simulink subsystem "thermal_subsystem_controller"  (R2023a)
settings: Solver=VariableStepAuto  StartTime=0.0  StopTime=10.0  RelTol=1e-3
undefined symbols (not defined in the file or in its folder): b_auxTCP_ACT, b_TCP_ACT, b_TCV_ACT, struct_auxTCP_ACT, struct_TCP_ACT, struct_TCV_ACT, struct_ThermalAct
libraries: simulink x4, eeGeneralControl x4, slpidlib x2
settings Model: Creator=daniel.harlander  LastModifiedBy=adrian.taveras
settings OptimizationCC: ReuseModelBlockBuffer=off

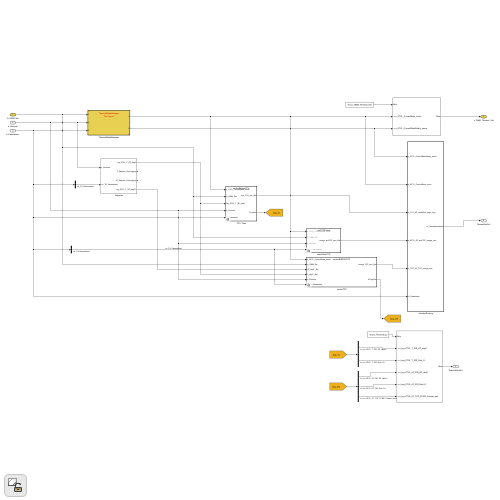
[thumbnail: Simulink's stored preview of the top-level diagram]
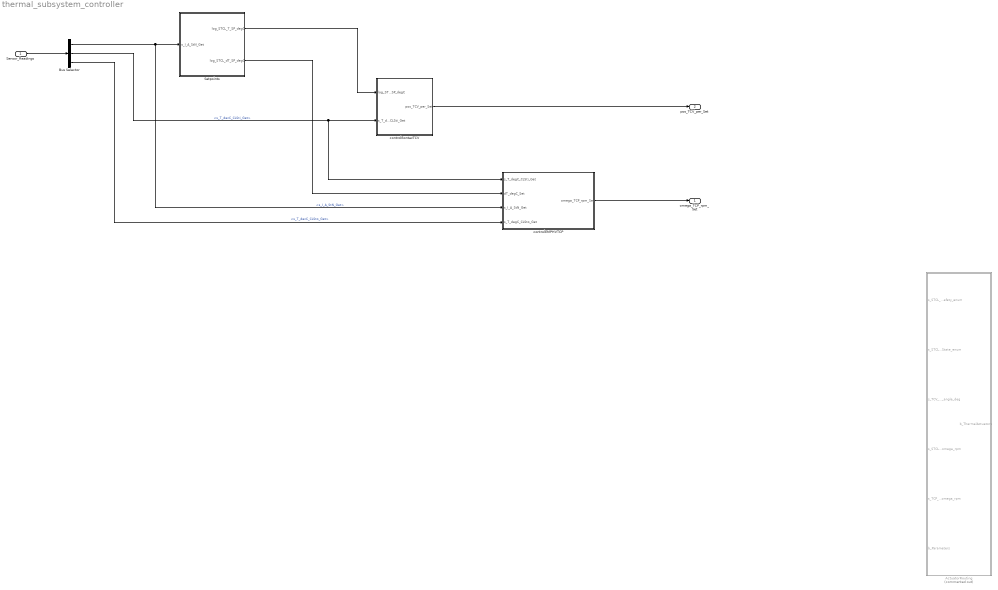
== system thermal_subsystem_controller ==
  Sensor_Readings : Inport
  ActuatorRouting : Subsystem  Commented=on  TreatAsAtomicUnit=on
      settings: RTWFcnNameOpts=Use subsystem name  RTWFileNameOpts=Use subsystem name
  Bus Selector : BusSelector  OutputSignals=s_I_A_StN_Get,s_T_decC_CLSti_Get,s_T_decC_CLSto_Get
  Setpoints : Subsystem
  controlBontazTCV : Subsystem  TreatAsAtomicUnit=on  VariantControl=variantConfig.TCV == VARIANT_TCV.BontazCAN
      settings: RTWFcnNameOpts=Use subsystem name  RTWFileNameOpts=Use subsystem name
  controlEMPHVTCP : Subsystem  TreatAsAtomicUnit=on  VariantControl=variantConfig.TCP == VARIANT_TCP.HVPump
  omega_TCP_rpm_Set : Outport
  pos_TCV_per_Set : Outport  Port=2
  wires:
  Setpoints/1(log_STCL_T_SP_degC) -> controlBontazTCV/1(log_STCL_T_SP_degC)
  Setpoints/2(log_STCL_dT_SP_degC) -> controlEMPHVTCP/2(dT_degC_Set)
  controlEMPHVTCP/1(omega_TCP_rpm_Set) -> omega_TCP_rpm_Set/1
  Sensor_Readings/1 -> Bus Selector/1
  Bus Selector/1 -> Setpoints/1(s_I_A_StN_Get), controlEMPHVTCP/3(s_I_A_StN_Get)  "<s_I_A_StN_Get>"
  Bus Selector/2 -> controlBontazTCV/2(s_T_decC_CLSti_Get), controlEMPHVTCP/1(s_T_degC_CLSti_Get)  "<s_T_decC_CLSti_Get>"
  Bus Selector/3 -> controlEMPHVTCP/4(s_T_degC_CLSto_Get)  "<s_T_decC_CLSto_Get>"
  controlBontazTCV/1(pos_TCV_per_Set) -> pos_TCV_per_Set/1

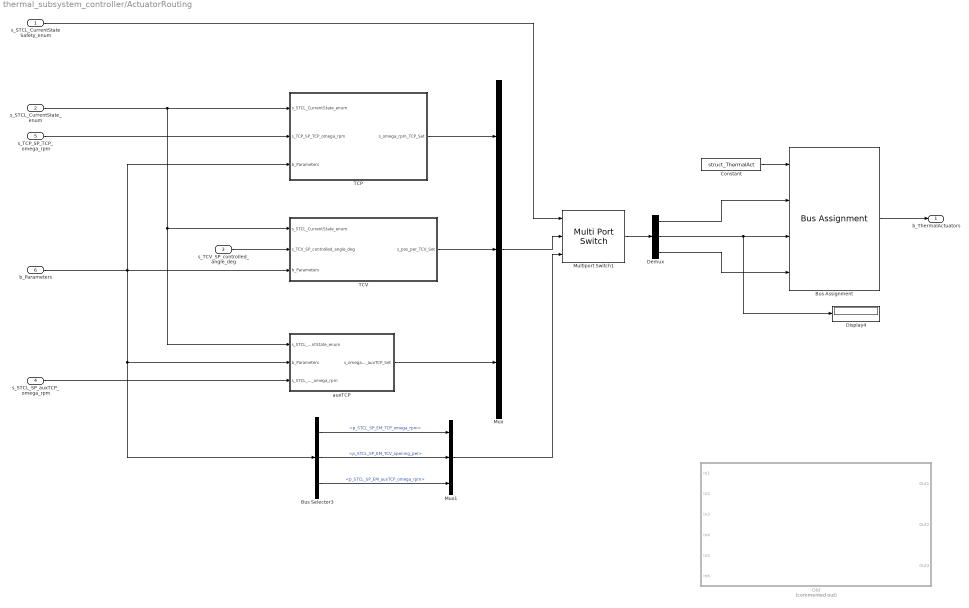
== system thermal_subsystem_controller/ActuatorRouting ==
  s_STCL_CurrentStateSafety_enum : Inport
  s_STCL_CurrentState_enum : Inport  Port=2
  s_TCV_SP_controlled_angle_deg : Inport  Port=3
  s_STCL_SP_auxTCP_omega_rpm : Inport  Port=4
  s_TCP_SP_TCP_omega_rpm : Inport  Port=5
  "b_Parameters  " : Inport  Port=6  OutDataTypeStr=Bus: Parameters
  Bus Assignment : BusAssignment  AssignedSignals=b_TCP_ACT.s_omega_rpm_TCP_Set,b_TCV_ACT.s_pos_per_TCV_Set,b_auxTCP_ACT.s_omega_rpm_auxTCP_Set
  Bus Selector3 : BusSelector  OutputSignals=b_TH_Parameters.b_STCL_Parameters.p_STCL_SP_EM_TCP_omega_rpm,b_TH_Parameters.b_STCL_Parameters.p_STCL_SP_EM_TCV_opening_per,b_TH_Parameters.b_STCL_Parameters.p_STCL_SP_EM_auxTCP_omega_rpm
  Constant : Constant  Value=struct_ThermalAct  OutDataTypeStr=Bus: ThermalAct
  Demux : Demux  Outputs=3
  Display4 : Display
  Multiport Switch1 : MultiPortSwitch  DataPortOrder=Specify indices  DataPortIndices={STCL_STATE_SAFETY.Safe, STCL_STATE_SAFETY.ESD_Off}  SaturateOnIntegerOverflow=off  InputSameDT=off
  Mux : Mux  Inputs=3
  Mux1 : Mux  Inputs=3
  Old : Subsystem  Commented=on
  TCP : Subsystem
  TCV : Subsystem
  auxTCP : Subsystem
  b_ThermalActuators : Outport
  wires:
  TCP/1(s_omega_rpm_TCP_Set) -> Mux/1
  s_TCP_SP_TCP_omega_rpm/1 -> TCP/2(s_TCP_SP_TCP_omega_rpm)
  TCV/1(s_pos_per_TCV_Set) -> Mux/2
  s_TCV_SP_controlled_angle_deg/1 -> TCV/2(s_TCV_SP_controlled_angle_deg)
  auxTCP/1(s_omega_rpm_auxTCP_Set) -> Mux/3
  s_STCL_SP_auxTCP_omega_rpm/1 -> auxTCP/3(s_STCL_SP_auxTCP_omega_rpm)
  Demux/3 -> Bus Assignment/4
  Demux/1 -> Bus Assignment/2
  Demux/2 -> Bus Assignment/3, Display4/1
  s_STCL_CurrentStateSafety_enum/1 -> Multiport Switch1/1
  Constant/1 -> Bus Assignment/1
  Bus Assignment/1 -> b_ThermalActuators/1
  s_STCL_CurrentState_enum/1 -> TCP/1(s_STCL_CurrentState_enum), TCV/1(s_STCL_CurrentState_enum), auxTCP/1(s_STCL_CurrentState_enum)
  Mux/1 -> Multiport Switch1/2
  Mux1/1 -> Multiport Switch1/3
  Multiport Switch1/1 -> Demux/1
  Bus Selector3/2 -> Mux1/2  "<p_STCL_SP_EM_TCV_opening_per>"
  Bus Selector3/3 -> Mux1/3  "<p_STCL_SP_EM_auxTCP_omega_rpm>"
  Bus Selector3/1 -> Mux1/1  "<p_STCL_SP_EM_TCP_omega_rpm>"
  "b_Parameters  "/1 -> TCV/3(b_Parameters), auxTCP/2(b_Parameters), Bus Selector3/1, TCP/3(b_Parameters)

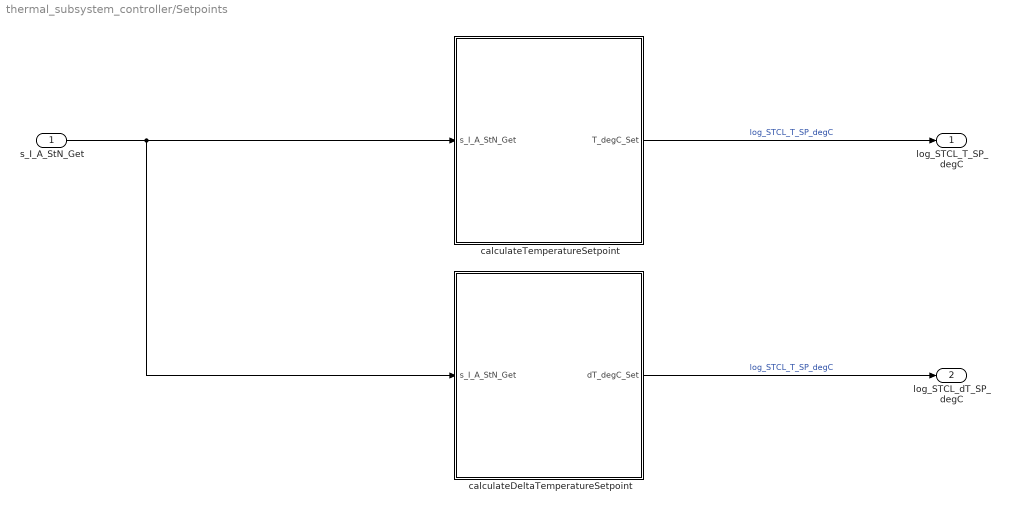
== system thermal_subsystem_controller/Setpoints ==
  s_I_A_StN_Get : Inport
  calculateDeltaTemperatureSetpoint : Subsystem  TreatAsAtomicUnit=on
      settings: RTWSystemCode=Nonreusable function  RTWFcnNameOpts=Use subsystem name  RTWFileNameOpts=Use subsystem name
  calculateTemperatureSetpoint : Subsystem  TreatAsAtomicUnit=on
      settings: RTWSystemCode=Nonreusable function  RTWFcnNameOpts=Use subsystem name  RTWFileNameOpts=Use subsystem name
  log_STCL_T_SP_degC : Outport
  log_STCL_dT_SP_degC : Outport  Port=2
  wires:
  calculateTemperatureSetpoint/1(T_degC_Set) -> log_STCL_T_SP_degC/1  "log_STCL_T_SP_degC"
  calculateDeltaTemperatureSetpoint/1(dT_degC_Set) -> log_STCL_dT_SP_degC/1  "log_STCL_T_SP_degC"
  s_I_A_StN_Get/1 -> calculateDeltaTemperatureSetpoint/1(s_I_A_StN_Get), calculateTemperatureSetpoint/1(s_I_A_StN_Get)

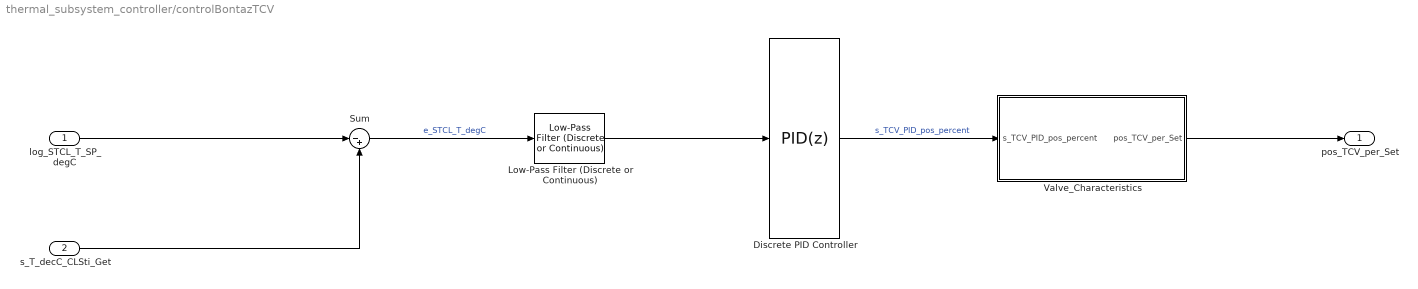
== system thermal_subsystem_controller/controlBontazTCV ==
  log_STCL_T_SP_degC : Inport
  s_T_decC_CLSti_Get : Inport  Port=2
  Discrete PID Controller : slpidlib/PID Controller  Controller=PID  Form=Parallel  TimeDomain=Discrete-time  UseExternalTs=off  SampleTime=-1  IntegratorMethod=Forward Euler  FilterMethod=Forward Euler  ControllerParametersSource=internal  P=2  I=0.75  UseKiTs=off  D=0  N=100  UseFilter=off  TunerSelectOption=Transfer Function Based (PID Tuner App)  InitialConditionSource=internal  InitialConditionForIntegrator=0  InitialConditionForFilter=0  DifferentiatorICPrevScaledInput=0  ExternalReset=none  TrackingMode=off  Kt=1  LimitOutput=on  SatLimitsSource=internal  UpperSaturationLimit=100  LowerSaturationLimit=0  LinearizeAsGain=on  AntiWindupMode=clamping  Kb=1  LimitIntegrator=off  UpperIntegratorSaturationLimit=inf  LowerIntegratorSaturationLimit=-inf  POutMin=[]  POutMax=[]  IOutMin=[]  IOutMax=[]  DOutMin=[]  DOutMax=[]  NOutMin=[]  NOutMax=[]  SumOutMin=[]  SumOutMax=[]  SaturationOutMin=[]  SaturationOutMax=[]  PParamMin=[]  PParamMax=[]  IParamMin=[]  IParamMax=[]  DParamMin=[]  DParamMax=[]  NParamMin=[]  NParamMax=[]  KbParamMin=[]  KbParamMax=[]  KtParamMin=[]  KtParamMax=[]  KbOutMin=[]  KbOutMax=[]  KtOutMin=[]  KtOutMax=[]  IntegratorOutMin=[]  IntegratorOutMax=[]  FilterOutMin=[]  FilterOutMax=[]  SumI1OutMin=[]  SumI1OutMax=[]  SumI2OutMin=[]  SumI2OutMax=[]  SumI3OutMin=[]  SumI3OutMax=[]  SumI4OutMin=[]  SumI4OutMax=[]  SumDOutMin=[]  SumDOutMax=[]  DifferentiatorOutMin=[]  DifferentiatorOutMax=[]  FilterDiffOutCoefMin=[]  FilterDiffOutCoefMax=[]  ReciprocalOutMin=[]  ReciprocalOutMax=[]  SumDenOutMin=[]  SumDenOutMax=[]  SumNumOutMin=[]  SumNumOutMax=[]  DivideOutMin=[]  DivideOutMax=[]  UdiffTsProdOutMin=[]  UdiffTsProdOutMax=[]  NTsProdOutMin=[]  NTsProdOutMax=[]  UintegralTsProdOutMin=[]  UintegralTsProdOutMax=[]  UngainTsProdOutMin=[]  UngainTsProdOutMax=[]  ClampingZeroOutDataTypeStr=Inherit: Inherit via back propagation  ClampingZeroOutMin=[]  ClampingZeroOutMax=[]  FilterDenConstantOutDataTypeStr=Inherit: Inherit via back propagation  FilterDenConstantOutMin=[]  FilterDenConstantOutMax=[]  PCopyOutDataTypeStr=Inherit: Inherit via back propagation  PCopyOutMin=[]  PCopyOutMax=[]  NCopyOutDataTypeStr=Inherit: Inherit via back propagation  NCopyOutMin=[]  NCopyOutMax=[]  IntegratorContinuousStateAttributes=''  IntegratorStateMustResolveToSignalObject=off  IntegratorRTWStateStorageClass=Auto  FilterContinuousStateAttributes=''  FilterStateMustResolveToSignalObject=off  FilterRTWStateStorageClass=Auto  ParallelPVariant=InternalParameters  IdealPVariant=Disabled  IVariant=InternalParameters  DVariant=InternalParameters  IntegratorVariant=Discrete  SatVariant=Enabled  AWVariant=DiscClampingParallel  PCopyVariant=Disabled  TRVariant=Disabled  FdbkBlocksVariant=Forward  IdealPFdbkVariant=Disabled  SatFdbkVariant=Disabled  DerivativeFilterVariant=Differentiator  NVariant=Passthrough  NCopyVariant=Disabled_SignalSpec  FilterICVariant=InternalICsDifferentiator  IntegratorICVariant=InternalICs  ExternalResetVariant=Disabled  TRSumVariant=Passthrough  SumFdbkVariant=Disabled  SumVariant=Sum_PID  TsampFilterVariant=InternalTs  TsampNgainVariant=Passthrough  TsampIntegralVariant=Disabled_SignalSpec  ExternalSaturationOutDataTypeStr=Inherit: Same as second input
      settings: LibrarySourceBlock=simulink/Discrete/Discrete PID Controller
  Low-Pass Filter (Discrete or Continuous) : eeGeneralControl/Low-Pass Filter (Discrete or Continuous)  K=1  T=1  B=inf  A=-inf  init_option=Inherited from block input  x0=0  Ts=-1
  Sum : Sum  Inputs=|-+
  Valve_Characteristics : Subsystem
  pos_TCV_per_Set : Outport
  wires:
  s_T_decC_CLSti_Get/1 -> Sum/2
  log_STCL_T_SP_degC/1 -> Sum/1
  Sum/1 -> Low-Pass Filter (Discrete or Continuous)/1  "e_STCL_T_degC"
  Low-Pass Filter (Discrete or Continuous)/1 -> Discrete PID Controller/1
  Discrete PID Controller/1 -> Valve_Characteristics/1(s_TCV_PID_pos_percent)  "s_TCV_PID_pos_percent"
  Valve_Characteristics/1(pos_TCV_per_Set) -> pos_TCV_per_Set/1

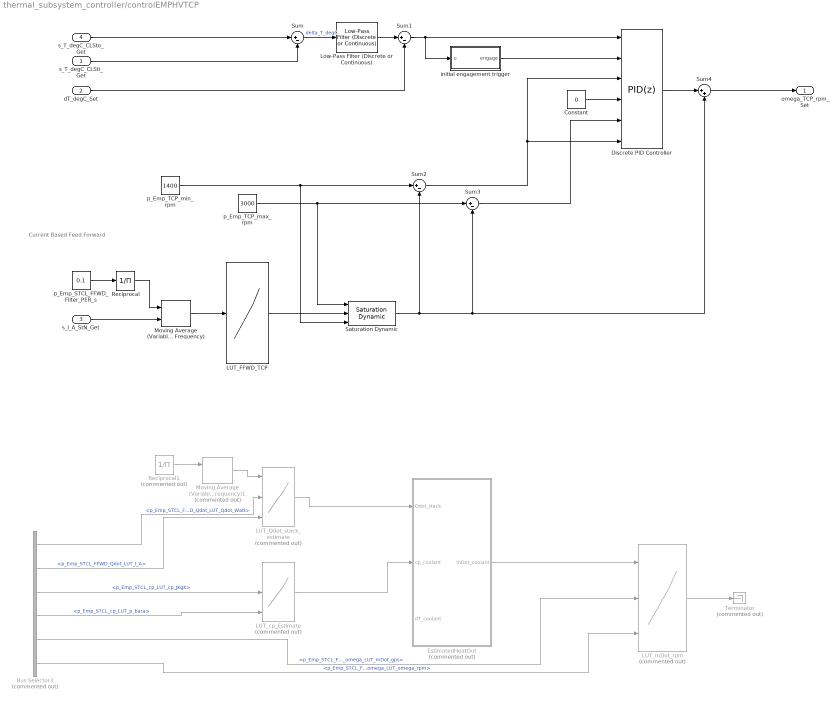
== system thermal_subsystem_controller/controlEMPHVTCP ==
  note: Current Based Feed Forward
  s_T_degC_CLSti_Get : Inport
  dT_degC_Set : Inport  Port=2
  s_I_A_StN_Get : Inport  Port=3
  s_T_degC_CLSto_Get : Inport  Port=4
  Bus Selector3 : BusSelector  Commented=on  OutputSignals=b_STCL_Parameters.p_Emp_STCL_FFWD_Qdot_LUT_Qdot_Watt,b_STCL_Parameters.p_Emp_STCL_FFWD_Qdot_LUT_I_A,b_STCL_Parameters.p_Emp_STCL_cp_LUT_cp_JKgK,b_STCL_Parameters.p_Emp_STCL_cp_LUT_p_bara,b_STCL_Parameters.p_Emp_STCL_FFWD_omega_LUT_mDot_gps,b_STCL_Parameters.p_Emp_STCL_FFWD_omega_LUT_omega_rpm
  Constant : Constant  Value=0  OutDataTypeStr=single
  Discrete PID Controller : slpidlib/PID Controller  Controller=PID  Form=Parallel  TimeDomain=Discrete-time  UseExternalTs=off  SampleTime=-1  IntegratorMethod=Forward Euler  FilterMethod=Forward Euler  ControllerParametersSource=internal  P=50  I=5  UseKiTs=off  D=0  N=100  UseFilter=off  TunerSelectOption=Transfer Function Based (PID Tuner App)  InitialConditionSource=external  InitialConditionForIntegrator=0  InitialConditionForFilter=0  DifferentiatorICPrevScaledInput=0  ExternalReset=rising  TrackingMode=off  Kt=1  LimitOutput=on  SatLimitsSource=external  UpperSaturationLimit=inf  LowerSaturationLimit=-inf  LinearizeAsGain=on  AntiWindupMode=clamping  Kb=1  LimitIntegrator=off  UpperIntegratorSaturationLimit=inf  LowerIntegratorSaturationLimit=-inf  POutMin=[]  POutMax=[]  IOutMin=[]  IOutMax=[]  DOutMin=[]  DOutMax=[]  NOutMin=[]  NOutMax=[]  SumOutMin=[]  SumOutMax=[]  SaturationOutMin=[]  SaturationOutMax=[]  PParamMin=[]  PParamMax=[]  IParamMin=[]  IParamMax=[]  DParamMin=[]  DParamMax=[]  NParamMin=[]  NParamMax=[]  KbParamMin=[]  KbParamMax=[]  KtParamMin=[]  KtParamMax=[]  KbOutMin=[]  KbOutMax=[]  KtOutMin=[]  KtOutMax=[]  IntegratorOutMin=[]  IntegratorOutMax=[]  FilterOutMin=[]  FilterOutMax=[]  SumI1OutMin=[]  SumI1OutMax=[]  SumI2OutMin=[]  SumI2OutMax=[]  SumI3OutMin=[]  SumI3OutMax=[]  SumI4OutMin=[]  SumI4OutMax=[]  SumDOutMin=[]  SumDOutMax=[]  DifferentiatorOutMin=[]  DifferentiatorOutMax=[]  FilterDiffOutCoefMin=[]  FilterDiffOutCoefMax=[]  ReciprocalOutMin=[]  ReciprocalOutMax=[]  SumDenOutMin=[]  SumDenOutMax=[]  SumNumOutMin=[]  SumNumOutMax=[]  DivideOutMin=[]  DivideOutMax=[]  UdiffTsProdOutMin=[]  UdiffTsProdOutMax=[]  NTsProdOutMin=[]  NTsProdOutMax=[]  UintegralTsProdOutMin=[]  UintegralTsProdOutMax=[]  UngainTsProdOutMin=[]  UngainTsProdOutMax=[]  ClampingZeroOutDataTypeStr=Inherit: Inherit via back propagation  ClampingZeroOutMin=[]  ClampingZeroOutMax=[]  FilterDenConstantOutDataTypeStr=Inherit: Inherit via back propagation  FilterDenConstantOutMin=[]  FilterDenConstantOutMax=[]  PCopyOutDataTypeStr=Inherit: Inherit via back propagation  PCopyOutMin=[]  PCopyOutMax=[]  NCopyOutDataTypeStr=Inherit: Inherit via back propagation  NCopyOutMin=[]  NCopyOutMax=[]  IntegratorContinuousStateAttributes=''  IntegratorStateMustResolveToSignalObject=off  IntegratorRTWStateStorageClass=Auto  FilterContinuousStateAttributes=''  FilterStateMustResolveToSignalObject=off  FilterRTWStateStorageClass=Auto  ParallelPVariant=InternalParameters  IdealPVariant=Disabled  IVariant=InternalParameters  DVariant=InternalParameters  IntegratorVariant=Discrete  SatVariant=External  AWVariant=DiscClampingParallel  PCopyVariant=Disabled  TRVariant=Disabled  FdbkBlocksVariant=Forward  IdealPFdbkVariant=Disabled  SatFdbkVariant=Disabled  DerivativeFilterVariant=Differentiator  NVariant=Passthrough  NCopyVariant=Disabled_SignalSpec  FilterICVariant=ExternalICs  IntegratorICVariant=ExternalICs  ExternalResetVariant=ExternalReset  TRSumVariant=Passthrough  SumFdbkVariant=Disabled  SumVariant=Sum_PID  TsampFilterVariant=InternalTs  TsampNgainVariant=Passthrough  TsampIntegralVariant=Disabled_SignalSpec  ExternalSaturationOutDataTypeStr=Inherit: Same as second input
      settings: LibrarySourceBlock=simulink/Discrete/Discrete PID Controller
  EstimatedHeatOut : MATLAB Function  Commented=on  TreatAsAtomicUnit=on
  LUT_FFWD_TCP : Lookup_n-D  NumberOfTableDimensions=1  BreakpointsForDimension1="[   0,  100,  199,  200,  250,  300,  350,  399,  400,  420,  450,  480,  500,  600]"  Table=[1400, 1400, 1600, 1800, 2200, 2600, 2800, 2900, 2900, 2900, 2900, 2900, 2900, 2900]  ExtrapMethod=Clip  UseLastTableValue=on  InternalRulePriority=Speed  RndMeth=Simplest
  LUT_Qdot_stack_estimate : Lookup_n-D  Commented=on  NumberOfTableDimensions=1  BreakpointsForDimension1Source=Input port  BreakpointsForDimension1=[-5:5]  TableSource=Input port  Table=tanh([-5:5])  ExtrapMethod=Clip  UseLastTableValue=on  InternalRulePriority=Speed  RndMeth=Simplest
      settings: InputPortMap=u0,p221,p5
  LUT_cp_Estimate : Lookup_n-D  Commented=on  NumberOfTableDimensions=1  BreakpointsForDimension1Source=Input port  BreakpointsForDimension1=[-5:5]  TableSource=Input port  Table=tanh([-5:5])  ExtrapMethod=Clip  UseLastTableValue=on  InternalRulePriority=Speed  RndMeth=Simplest
      settings: InputPortMap=u0,p221,p5
  LUT_mDot_rpm : Lookup_n-D  Commented=on  NumberOfTableDimensions=1  BreakpointsForDimension1Source=Input port  BreakpointsForDimension1=[-5:5]  TableSource=Input port  Table=tanh([-5:5])  ExtrapMethod=Clip  UseLastTableValue=on  InternalRulePriority=Speed  RndMeth=Simplest
      settings: InputPortMap=u0,p221,p5
  Low-Pass Filter (Discrete or Continuous) : eeGeneralControl/Low-Pass Filter (Discrete or Continuous)  K=1  T=1  B=inf  A=-inf  init_option=Inherited from block input  x0=0  Ts=-1
  Moving Average (Variable Frequency) : eeGeneralControl/Moving Average (Variable Frequency)  VariantControl=Variant1  LabelModeActiveChoice=Discrete  f0=100  fmin=0.1  x0=0  BufferSize=8192  Ts=-1
      settings: LibrarySourceBlock=|
      | ee_sl_lib/General Control/Moving Average
      | (Variable Frequency)
  Moving Average (Variable Frequency)1 : eeGeneralControl/Moving Average (Variable Frequency)  Commented=on  VariantControl=Variant1  LabelModeActiveChoice=Discrete  f0=100  fmin=0.1  x0=0  BufferSize=8192  Ts=-1
      settings: LibrarySourceBlock=|
      | ee_sl_lib/General Control/Moving Average
      | (Variable Frequency)
  Reciprocal : Product  Inputs=/
  Reciprocal1 : Product  Commented=on  Inputs=/
  Saturation Dynamic : simulink/Discontinuities/Saturation Dynamic  OutMin=[]  OutMax=[]  OutDataTypeStr=Inherit: Same as second input  OutDataType=fixdt(1, 16)  OutScaling=2^-10  DoSatur=off
  Sum{,1..3} (4 alike) : Sum  Inputs=|+-
  Sum4 : Sum  Inputs=|++
  Terminator : Terminator  Commented=on
  initial engagement trigger : Subsystem
  p_Emp_STCL_FFWD_Filter_PER_s : Constant  Value=0.1
  p_Emp_TCP_max_rpm : Constant  Value=3000
  p_Emp_TCP_min_rpm : Constant  Value=1400
  omega_TCP_rpm_Set : Outport
  wires:
  initial engagement trigger/1(engage) -> Discrete PID Controller/2
  LUT_mDot_rpm/1 -> Terminator/1
  Bus Selector3/3 -> LUT_cp_Estimate/2  "<p_Emp_STCL_cp_LUT_cp_JKgK>"
  Bus Selector3/4 -> LUT_cp_Estimate/3  "<p_Emp_STCL_cp_LUT_p_bara>"
  LUT_cp_Estimate/1 -> EstimatedHeatOut/2(cp_coolant)
  Bus Selector3/6 -> LUT_mDot_rpm/3  "<p_Emp_STCL_FFWD_omega_LUT_omega_rpm>"
  Bus Selector3/5 -> LUT_mDot_rpm/2  "<p_Emp_STCL_FFWD_omega_LUT_mDot_gps>"
  Bus Selector3/2 -> LUT_Qdot_stack_estimate/3  "<p_Emp_STCL_FFWD_Qdot_LUT_I_A>"
  Bus Selector3/1 -> LUT_Qdot_stack_estimate/2  "<p_Emp_STCL_FFWD_Qdot_LUT_Qdot_Watt>"
  Reciprocal1/1 -> Moving Average (Variable Frequency)1/1
  Moving Average (Variable Frequency)1/1 -> LUT_Qdot_stack_estimate/1
  EstimatedHeatOut/1(mDot_coolant) -> LUT_mDot_rpm/1
  LUT_Qdot_stack_estimate/1 -> EstimatedHeatOut/1(Qdot_stack)
  Discrete PID Controller/1 -> Sum4/1
  s_T_degC_CLSti_Get/1 -> Sum/2
  p_Emp_TCP_min_rpm/1 -> Saturation Dynamic/3, Sum2/1
  s_T_degC_CLSto_Get/1 -> Sum/1
  Low-Pass Filter (Discrete or Continuous)/1 -> Sum1/1
  Sum1/1 -> Discrete PID Controller/1, initial engagement trigger/1(u)
  p_Emp_TCP_max_rpm/1 -> Sum3/1, Saturation Dynamic/1
  Constant/1 -> Discrete PID Controller/4
  Sum/1 -> Low-Pass Filter (Discrete or Continuous)/1  "delta_T_degC"
  dT_degC_Set/1 -> Sum1/2
  Moving Average (Variable Frequency)/1 -> LUT_FFWD_TCP/1
  s_I_A_StN_Get/1 -> Moving Average (Variable Frequency)/2
  LUT_FFWD_TCP/1 -> Saturation Dynamic/2
  Saturation Dynamic/1 -> Sum4/2, Sum3/2, Sum2/2
  Sum2/1 -> Discrete PID Controller/6, Discrete PID Controller/3
  Sum3/1 -> Discrete PID Controller/5
  Sum4/1 -> omega_TCP_rpm_Set/1
  p_Emp_STCL_FFWD_Filter_PER_s/1 -> Reciprocal/1
  Reciprocal/1 -> Moving Average (Variable Frequency)/1

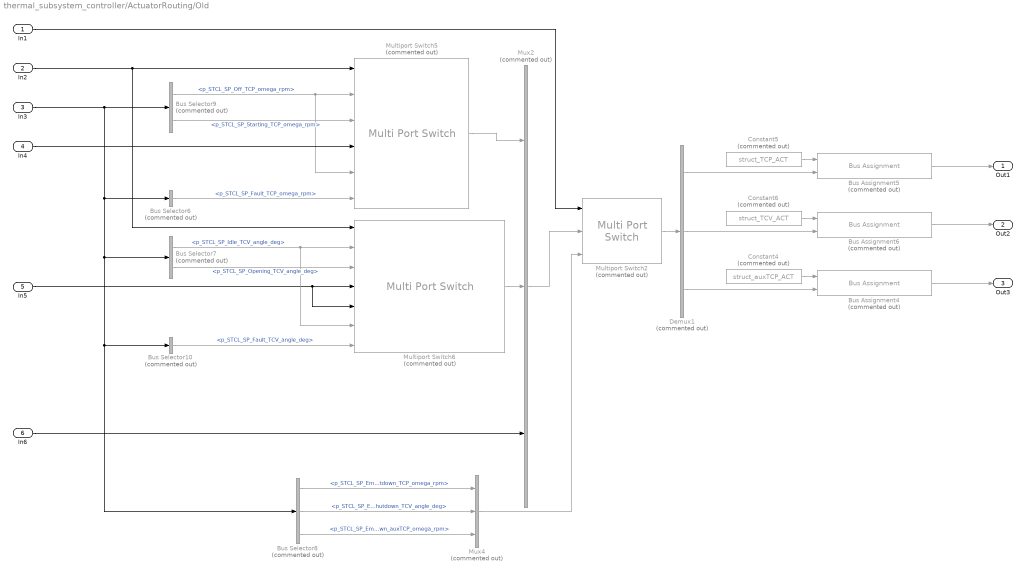
== system thermal_subsystem_controller/ActuatorRouting/Old ==
  In1 : Inport
  In2 : Inport  Port=2
  In3 : Inport  Port=3
  In4 : Inport  Port=4
  In5 : Inport  Port=5
  In6 : Inport  Port=6
  Bus Assignment4 : BusAssignment  Commented=on  AssignedSignals=s_omega_rpm_auxTCP_Set
  Bus Assignment5 : BusAssignment  Commented=on  AssignedSignals=s_omega_rpm_TCP_Set
  Bus Assignment6 : BusAssignment  Commented=on  AssignedSignals=s_pos_deg_TCV_Set
  Bus Selector10 : BusSelector  Commented=on  OutputSignals=b_TH_Parameters.b_STCL_Parameters.p_STCL_SP_Fault_TCV_angle_deg
  Bus Selector6 : BusSelector  Commented=on  OutputSignals=b_TH_Parameters.b_STCL_Parameters.p_STCL_SP_Fault_TCP_omega_rpm
  Bus Selector7 : BusSelector  Commented=on  OutputSignals=b_TH_Parameters.b_STCL_Parameters.p_STCL_SP_Idle_TCV_angle_deg,b_TH_Parameters.b_STCL_Parameters.p_STCL_SP_Opening_TCV_angle_deg
  Bus Selector8 : BusSelector  Commented=on  OutputSignals=b_TH_Parameters.b_STCL_Parameters.p_STCL_SP_EmergencyShutdown_TCP_omega_rpm,b_TH_Parameters.b_STCL_Parameters.p_STCL_SP_EmergencyShutdown_TCV_angle_deg,b_TH_Parameters.b_STCL_Parameters.p_STCL_SP_EmergencyShutdown_auxTCP_omega_rpm
  Bus Selector9 : BusSelector  Commented=on  OutputSignals=b_TH_Parameters.b_STCL_Parameters.p_STCL_SP_Off_TCP_omega_rpm,b_TH_Parameters.b_STCL_Parameters.p_STCL_SP_Starting_TCP_omega_rpm
  Constant4 : Constant  Commented=on  Value=struct_auxTCP_ACT  OutDataTypeStr=Bus: auxTCP_ACT
  Constant5 : Constant  Commented=on  Value=struct_TCP_ACT  OutDataTypeStr=Bus: TCP_ACT
  Constant6 : Constant  Commented=on  Value=struct_TCV_ACT  OutDataTypeStr=Bus: TCV_ACT
  Demux1 : Demux  Commented=on  Outputs=3
  Multiport Switch2 : MultiPortSwitch  Commented=on  DataPortOrder=Specify indices  DataPortIndices={STCL_STATE_SAFETY.Safe, STCL_STATE_SAFETY.EmergencyShutdown}  SaturateOnIntegerOverflow=off  InputSameDT=off
  Multiport Switch5 : MultiPortSwitch  Commented=on  DataPortOrder=Specify indices  DataPortIndices=|  SaturateOnIntegerOverflow=off  InputSameDT=off
      | {[STCL_STATE.Off,
      | STCL_STATE.OpeningTCV],
      | STCL_STATE.StartingTCP,
      | [STCL_STATE.Operational,
      | STCL_STATE.ShutdownCooling],
      | [STCL_STATE.StoppingTCP,
      | STCL_STATE.ClosingTCV],
      | STCL_STATE.Fault}
  Multiport Switch6 : MultiPortSwitch  Commented=on  DataPortOrder=Specify indices  DataPortIndices=|  SaturateOnIntegerOverflow=off  InputSameDT=off
      | {STCL_STATE.Off,
      | [STCL_STATE.OpeningTCV,
      | STCL_STATE.StartingTCP],
      | [STCL_STATE.Operational,
      | STCL_STATE.ShutdownCooling],
      | STCL_STATE.StoppingTCP,
      | STCL_STATE.ClosingTCV,
      | STCL_STATE.Fault}
  Mux2 : Mux  Commented=on  Inputs=3
  Mux4 : Mux  Commented=on  Inputs=3
  Out1 : Outport
  Out2 : Outport  Port=2
  Out3 : Outport  Port=3
  wires:
  Bus Selector6/1 -> Multiport Switch5/6  "<p_STCL_SP_Fault_TCP_omega_rpm>"
  In5/1 -> Multiport Switch6/5, Multiport Switch6/4
  Demux1/1 -> Bus Assignment5/2
  Bus Selector7/2 -> Multiport Switch6/3  "<p_STCL_SP_Opening_TCV_angle_deg>"
  Mux2/1 -> Multiport Switch2/2
  Constant6/1 -> Bus Assignment6/1
  Multiport Switch2/1 -> Demux1/1
  Bus Selector9/2 -> Multiport Switch5/3  "<p_STCL_SP_Starting_TCP_omega_rpm>"
  Multiport Switch5/1 -> Mux2/1
  Demux1/3 -> Bus Assignment4/2
  Bus Assignment4/1 -> Out3/1
  In2/1 -> Multiport Switch6/1, Multiport Switch5/1
  Bus Selector8/2 -> Mux4/2  "<p_STCL_SP_EmergencyShutdown_TCV_angle_deg>"
  Multiport Switch6/1 -> Mux2/2
  Bus Selector7/1 -> Multiport Switch6/6, Multiport Switch6/2  "<p_STCL_SP_Idle_TCV_angle_deg>"
  Bus Selector9/1 -> Multiport Switch5/5, Multiport Switch5/2  "<p_STCL_SP_Off_TCP_omega_rpm>"
  Bus Selector8/1 -> Mux4/1  "<p_STCL_SP_EmergencyShutdown_TCP_omega_rpm>"
  Bus Selector8/3 -> Mux4/3  "<p_STCL_SP_EmergencyShutdown_auxTCP_omega_rpm>"
  Constant5/1 -> Bus Assignment5/1
  In3/1 -> Bus Selector9/1, Bus Selector6/1, Bus Selector7/1, Bus Selector10/1, Bus Selector8/1
  In6/1 -> Mux2/3
  Mux4/1 -> Multiport Switch2/3
  Bus Selector10/1 -> Multiport Switch6/7  "<p_STCL_SP_Fault_TCV_angle_deg>"
  Demux1/2 -> Bus Assignment6/2
  Bus Assignment5/1 -> Out1/1
  Constant4/1 -> Bus Assignment4/1
  In4/1 -> Multiport Switch5/4
  In1/1 -> Multiport Switch2/1
  Bus Assignment6/1 -> Out2/1

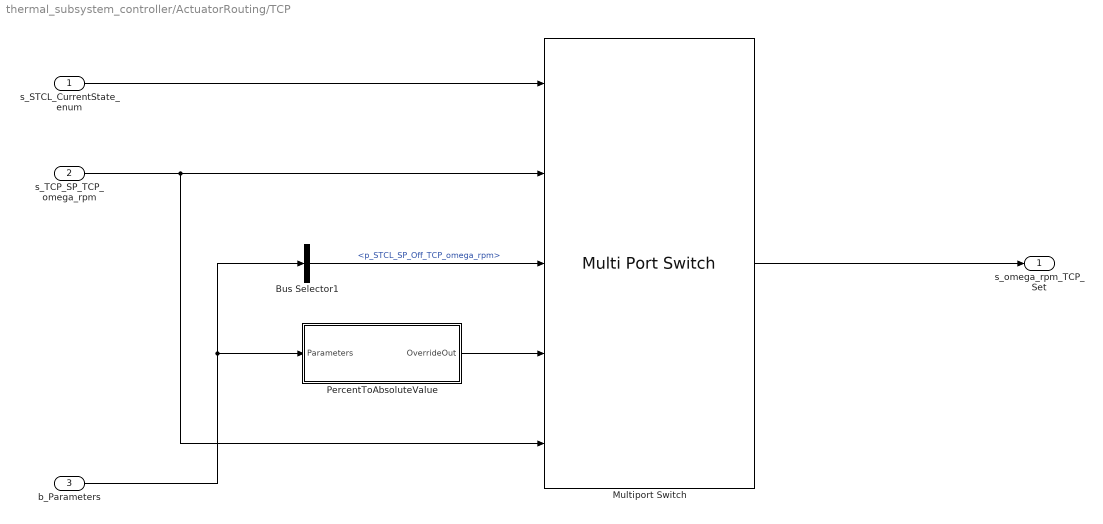
== system thermal_subsystem_controller/ActuatorRouting/TCP ==
  s_STCL_CurrentState_enum : Inport  OutDataTypeStr=Enum: STCL_STATE
  s_TCP_SP_TCP_omega_rpm : Inport  Port=2
  b_Parameters : Inport  Port=3  OutDataTypeStr=Bus: Parameters
  Bus Selector1 : BusSelector  OutputSignals=b_TH_Parameters.b_STCL_Parameters.p_STCL_SP_Off_TCP_omega_rpm
  Multiport Switch : MultiPortSwitch  DataPortOrder=Specify indices  DataPortIndices={STCL_STATE.NormalOperationMode1, [STCL_STATE.Off, STCL_STATE.TurningOff], STCL_STATE.MaintenanceOverride}  DataPortForDefault=Additional data port  DiagnosticForDefault=None  SaturateOnIntegerOverflow=off  InputSameDT=off
  PercentToAbsoluteValue : Subsystem  Variant=on  VariantControl=Choice  VariantActivationTime=startup
  s_omega_rpm_TCP_Set : Outport
  wires:
  Multiport Switch/1 -> s_omega_rpm_TCP_Set/1
  Bus Selector1/1 -> Multiport Switch/3  "<p_STCL_SP_Off_TCP_omega_rpm>"
  PercentToAbsoluteValue/1(OverrideOut) -> Multiport Switch/4
  s_STCL_CurrentState_enum/1 -> Multiport Switch/1
  s_TCP_SP_TCP_omega_rpm/1 -> Multiport Switch/2, Multiport Switch/5
  b_Parameters/1 -> PercentToAbsoluteValue/1(Parameters), Bus Selector1/1

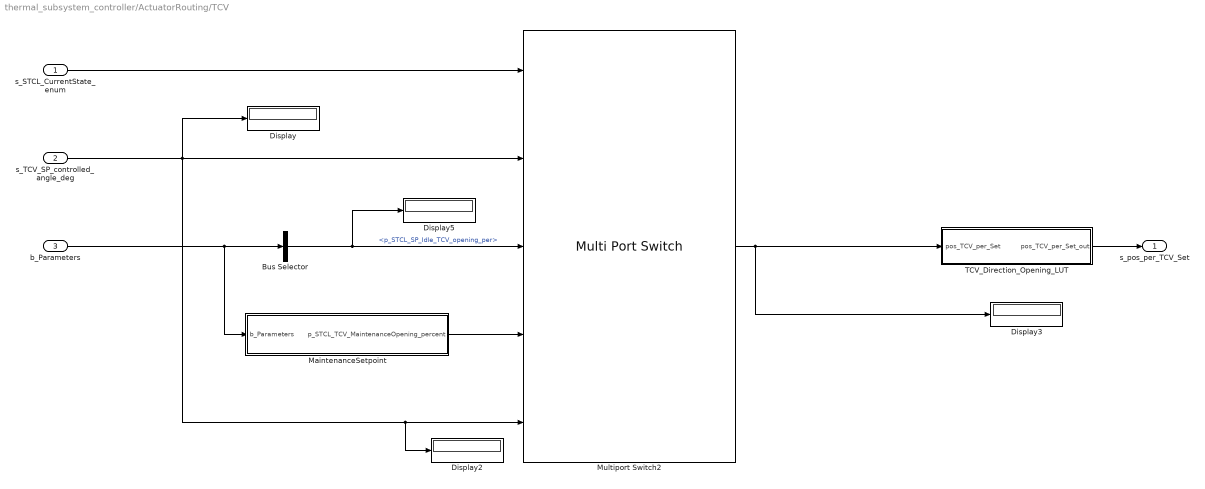
== system thermal_subsystem_controller/ActuatorRouting/TCV ==
  s_STCL_CurrentState_enum : Inport  OutDataTypeStr=Enum: STCL_STATE
  s_TCV_SP_controlled_angle_deg : Inport  Port=2
  b_Parameters : Inport  Port=3  OutDataTypeStr=Bus: Parameters
  Bus Selector : BusSelector  OutputSignals=b_TH_Parameters.b_STCL_Parameters.p_STCL_SP_Idle_TCV_opening_per
  Display{,2..3,5} (4 alike) : Display
  MaintenanceSetpoint : Subsystem
  Multiport Switch2 : MultiPortSwitch  DataPortOrder=Specify indices  DataPortIndices={STCL_STATE.NormalOperationMode1, [STCL_STATE.Off, STCL_STATE.TurningOff], STCL_STATE.MaintenanceOverride}  DataPortForDefault=Additional data port  DiagnosticForDefault=None  SaturateOnIntegerOverflow=off  InputSameDT=off
  TCV_Direction_Opening_LUT : Subsystem  Variant=on  VariantActivationTime=startup
  s_pos_per_TCV_Set : Outport
  wires:
  MaintenanceSetpoint/1(p_STCL_TCV_MaintenanceOpening_percent) -> Multiport Switch2/4
  TCV_Direction_Opening_LUT/1(pos_TCV_per_Set_out) -> s_pos_per_TCV_Set/1
  Bus Selector/1 -> Display5/1, Multiport Switch2/3  "<p_STCL_SP_Idle_TCV_opening_per>"
  Multiport Switch2/1 -> TCV_Direction_Opening_LUT/1(pos_TCV_per_Set), Display3/1
  b_Parameters/1 -> Bus Selector/1, MaintenanceSetpoint/1(b_Parameters)
  s_TCV_SP_controlled_angle_deg/1 -> Multiport Switch2/5, Display2/1, Multiport Switch2/2, Display/1
  s_STCL_CurrentState_enum/1 -> Multiport Switch2/1

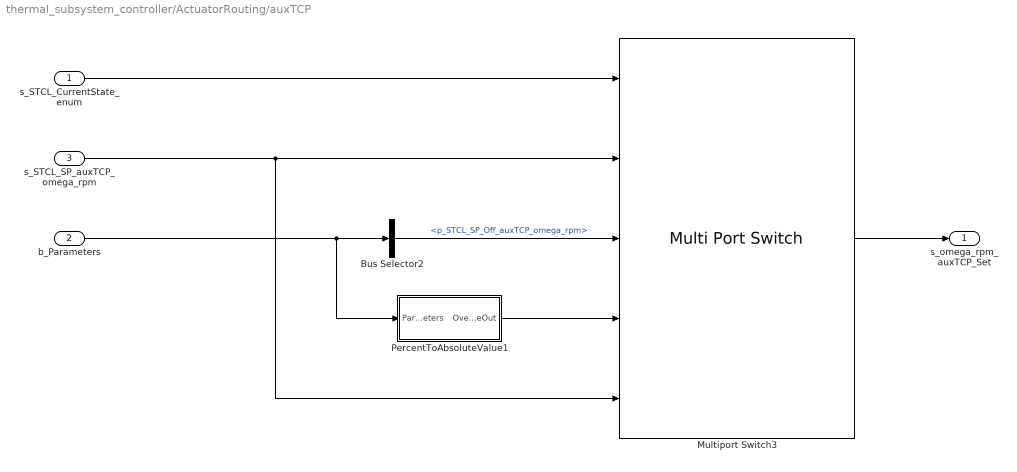
== system thermal_subsystem_controller/ActuatorRouting/auxTCP ==
  s_STCL_CurrentState_enum : Inport  OutDataTypeStr=Enum: STCL_STATE
  b_Parameters : Inport  Port=2
  s_STCL_SP_auxTCP_omega_rpm : Inport  Port=3
  Bus Selector2 : BusSelector  OutputSignals=b_TH_Parameters.b_STCL_Parameters.p_STCL_SP_Off_auxTCP_omega_rpm
  Multiport Switch3 : MultiPortSwitch  DataPortOrder=Specify indices  DataPortIndices={STCL_STATE.NormalOperationMode1, [STCL_STATE.Off, STCL_STATE.TurningOff], STCL_STATE.MaintenanceOverride}  DataPortForDefault=Additional data port  DiagnosticForDefault=None  SaturateOnIntegerOverflow=off  InputSameDT=off
  PercentToAbsoluteValue1 : Subsystem
  s_omega_rpm_auxTCP_Set : Outport
  wires:
  PercentToAbsoluteValue1/1(OverrideOut) -> Multiport Switch3/4
  s_STCL_CurrentState_enum/1 -> Multiport Switch3/1
  Bus Selector2/1 -> Multiport Switch3/3  "<p_STCL_SP_Off_auxTCP_omega_rpm>"
  b_Parameters/1 -> Bus Selector2/1, PercentToAbsoluteValue1/1(Parameters)
  s_STCL_SP_auxTCP_omega_rpm/1 -> Multiport Switch3/2, Multiport Switch3/5
  Multiport Switch3/1 -> s_omega_rpm_auxTCP_Set/1

== system thermal_subsystem_controller/Setpoints/calculateDeltaTemperatureSetpoint ==
  s_I_A_StN_Get : Inport
  1-D Lookup Table1 : Lookup_n-D  NumberOfTableDimensions=1  BreakpointsForDimension1="[0   50   100   150   200   250   300   350   400   425   450   475   500]"  BreakpointsForDimension2Source=Input port  Table="[ 8, 8,    8,    8,     8,    8,    8,    8,     9,   10,   11,   12,   13]"  ExtrapMethod=Clip  InternalRulePriority=Speed  RndMeth=Simplest
  dT_degC_Set : Outport
  wires:
  s_I_A_StN_Get/1 -> 1-D Lookup Table1/1
  1-D Lookup Table1/1 -> dT_degC_Set/1

== system thermal_subsystem_controller/Setpoints/calculateTemperatureSetpoint ==
  s_I_A_StN_Get : Inport
  1-D Lookup Table1 : Lookup_n-D  NumberOfTableDimensions=1  BreakpointsForDimension1="[0   50   100   150   200   250   300   350   400   425   450   475   500]"  BreakpointsForDimension2Source=Input port  Table="[58, 58,   62,   64,   66,   69,   72,  73,   73,   73,   73,   73,   73]"  ExtrapMethod=Clip  InternalRulePriority=Speed  RndMeth=Simplest
  T_degC_Set : Outport
  wires:
  s_I_A_StN_Get/1 -> 1-D Lookup Table1/1
  1-D Lookup Table1/1 -> T_degC_Set/1

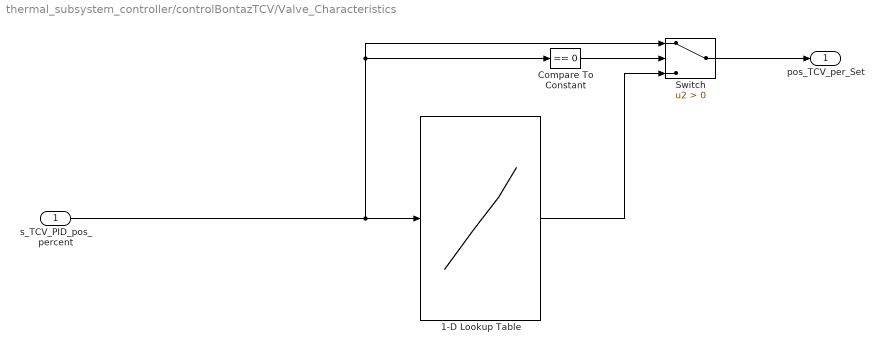
== system thermal_subsystem_controller/controlBontazTCV/Valve_Characteristics ==
  s_TCV_PID_pos_percent : Inport
  1-D Lookup Table : Lookup_n-D  NumberOfTableDimensions=1  BreakpointsForDimension1="[5  10  70  73 80 100]"  Table="[0  2   91  95 99 100]"  InternalRulePriority=Speed  RndMeth=Simplest
  Compare To Constant : simulink/Logic and Bit Operations/Compare To Constant  relop===  const=0  OutDataTypeStr=boolean
  Switch : Switch  Criteria=u2 > Threshold  SaturateOnIntegerOverflow=off  InputSameDT=off
  pos_TCV_per_Set : Outport
  wires:
  Switch/1 -> pos_TCV_per_Set/1
  1-D Lookup Table/1 -> Switch/3
  Compare To Constant/1 -> Switch/2
  s_TCV_PID_pos_percent/1 -> Compare To Constant/1, Switch/1, 1-D Lookup Table/1

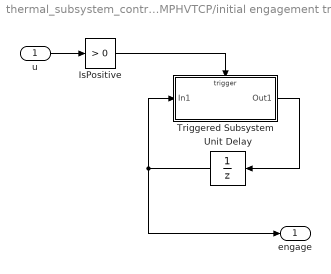
== system thermal_subsystem_controller/controlEMPHVTCP/initial engagement trigger ==
  u : Inport
  IsPositive : simulink/Logic and Bit Operations/Compare To Zero  relop=>  OutDataTypeStr=boolean
      settings: LibrarySourceBlock=|
      | simulink/Quick Insert/Logic and Bit
      | Operations/IsPositive
  Triggered Subsystem : Subsystem  TreatAsAtomicUnit=on
  Unit Delay : UnitDelay  SampleTime=-1  HasFrameUpgradeWarning=on
  engage : Outport
  wires:
  u/1 -> IsPositive/1
  IsPositive/1 -> Triggered Subsystem/Trigger
  Unit Delay/1 -> engage/1, Triggered Subsystem/1(In1)
  Triggered Subsystem/1(Out1) -> Unit Delay/1

== system thermal_subsystem_controller/ActuatorRouting/TCP/PercentToAbsoluteValue ==
  Parameters : Inport
  PercentToAbsoluteValueHVPump : Subsystem  TreatAsAtomicUnit=on  VariantControl=variantConfig.TCP == VARIANT_TCP.HVPump
  PercentToAbsoluteValueValeo : Subsystem  TreatAsAtomicUnit=on  VariantControl=variantConfig.TCP == VARIANT_TCP.ValeoSPumpPS100
  OverrideOut : Outport

== system thermal_subsystem_controller/ActuatorRouting/TCV/MaintenanceSetpoint ==
  b_Parameters : Inport  OutDataTypeStr=Bus: Parameters
  Bus Selector4 : BusSelector  OutputSignals=b_SERVICE_Parameters.p_STCL_TCV_MaxVentingOpening_percent,b_SERVICE_Parameters.p_STCL_TCV_VentingOpening_percent,b_SERVICE_Parameters.p_STCL_TCV_MinVentingOpening_percent
  Saturation Dynamic : simulink/Discontinuities/Saturation Dynamic  OutMin=[]  OutMax=[]  OutDataTypeStr=Inherit: Same as second input  OutDataType=fixdt(1, 16)  OutScaling=2^-10  DoSatur=off
  p_STCL_TCV_MaintenanceOpening_percent : Outport
  wires:
  Bus Selector4/1 -> Saturation Dynamic/1  "<p_STCL_TCV_MaxVentingOpening_percent>"
  Saturation Dynamic/1 -> p_STCL_TCV_MaintenanceOpening_percent/1
  Bus Selector4/3 -> Saturation Dynamic/3  "<p_STCL_TCV_MinVentingOpening_percent>"
  b_Parameters/1 -> Bus Selector4/1
  Bus Selector4/2 -> Saturation Dynamic/2  "<p_STCL_TCV_VentingOpening_percent>"

== system thermal_subsystem_controller/ActuatorRouting/TCV/TCV_Direction_Opening_LUT ==
  note: 1) Add Subsystem or Model blocks as valid variant choices.
      | 2) You cannot connect blocks at this level. At simulation, connectivity is automatically
      | determined, based on the active variant and port name matching.
  pos_TCV_per_Set : Inport
  Open_Leads_To_Cooling : Subsystem  TreatAsAtomicUnit=on  VariantControl=variantConfig.TCVDirection == VARIANT_TCVDirection.OPEN_IS_COOLING
  Open_Leads_To_Heating : Subsystem  TreatAsAtomicUnit=on  VariantControl=variantConfig.TCVDirection == VARIANT_TCVDirection.OPEN_IS_HEATING
  pos_TCV_per_Set_out : Outport

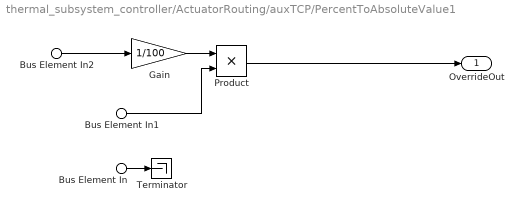
== system thermal_subsystem_controller/ActuatorRouting/auxTCP/PercentToAbsoluteValue1 ==
  Bus Element In : Inport  PortName=Parameters  Element=b_TH_Parameters.b_STCL_Parameters.p_auxTCP_min_rpm
  Bus Element In1 : Inport  PortName=Parameters  Element=b_TH_Parameters.b_STCL_Parameters.p_auxTCP_max_rpm
  Bus Element In2 : Inport  PortName=Parameters  Element=b_SERVICE_Parameters.p_STCL_auxTCP_VentingOmega_percent
  Gain : Gain  Gain=1/100
  Product : Product
  Terminator : Terminator
  OverrideOut : Outport
  wires:
  Bus Element In2/1 -> Gain/1
  Bus Element In/1 -> Terminator/1
  Gain/1 -> Product/1
  Bus Element In1/1 -> Product/2
  Product/1 -> OverrideOut/1

== system thermal_subsystem_controller/controlEMPHVTCP/initial engagement trigger/Triggered Subsystem ==
  In1 : Inport
  Trigger : TriggerPort  VariantControl=(inherit)
  Constant : Constant  OutDataTypeStr=boolean
  Switch : Switch  Criteria=u2 > Threshold  SaturateOnIntegerOverflow=off  InputSameDT=off
  Out1 : Outport
  wires:
  Constant/1 -> Switch/3
  In1/1 -> Switch/1, Switch/2
  Switch/1 -> Out1/1

== system thermal_subsystem_controller/ActuatorRouting/TCP/PercentToAbsoluteValue/PercentToAbsoluteValueHVPump ==
  Bus Element In1 : Inport  PortName=Parameters  Element=b_TH_Parameters.b_STCL_Parameters.p_Emp_TCP_max_rpm
  Bus Element In2 : Inport  PortName=Parameters  Element=b_SERVICE_Parameters.p_STCL_TCP_VentingOmega_percent
  Gain : Gain  Gain=1/100
  Product : Product
  OverrideOut : Outport
  wires:
  Bus Element In2/1 -> Gain/1
  Gain/1 -> Product/1
  Bus Element In1/1 -> Product/2
  Product/1 -> OverrideOut/1

== system thermal_subsystem_controller/ActuatorRouting/TCP/PercentToAbsoluteValue/PercentToAbsoluteValueValeo ==
  Bus Element In1 : Inport  PortName=Parameters  Element=b_TH_Parameters.b_STCL_Parameters.p_Vlo_TCP_max_rpm
  Bus Element In2 : Inport  PortName=Parameters  Element=b_SERVICE_Parameters.p_STCL_TCP_VentingOmega_percent
  Gain : Gain  Gain=1/100
  Product : Product
  OverrideOut : Outport
  wires:
  Product/1 -> OverrideOut/1
  Bus Element In1/1 -> Product/2
  Gain/1 -> Product/1
  Bus Element In2/1 -> Gain/1

== system thermal_subsystem_controller/ActuatorRouting/TCV/TCV_Direction_Opening_LUT/Open_Leads_To_Cooling ==
  pos_TCV_per_Set : Inport
  pos_TCV_per_Set_out : Outport
  wires:
  pos_TCV_per_Set/1 -> pos_TCV_per_Set_out/1

== system thermal_subsystem_controller/ActuatorRouting/TCV/TCV_Direction_Opening_LUT/Open_Leads_To_Heating ==
  pos_TCV_per_Set : Inport
  Add : Sum  Inputs=+-
  Constant : Constant  Value=100  OutDataTypeStr=single
  pos_TCV_per_Set_out : Outport
  wires:
  Add/1 -> pos_TCV_per_Set_out/1
  pos_TCV_per_Set/1 -> Add/2
  Constant/1 -> Add/1

== matlab function thermal_subsystem_controller/controlEMPHVTCP/EstimatedHeatOut ==
  data: Qdot_stack input; mDot_coolant output; cp_coolant input; dT_coolant input
function mDot_coolant = fcn(Qdot_stack, cp_coolant, dT_coolant)

mDot_coolant = Qdot_stack / (cp_coolant * dT_coolant);
